simulink model "FullSystemNoFilters"  (R2023b)
settings: Solver=ode4  StartTime=0.0  StopTime=5  FixedStep=0.002  RelTol=1e-3  AbsTol=1e-6  EnableMultiTasking=on
undefined symbols (not defined in the file): den, kd, ki, kp, num, VMAX_DAC
settings Model: ExtModeTrigDuration=10000  Creator=MLevis  LastModifiedBy=JTayl
settings SolverCC: AutoScaleAbsTol=off  AlgebraicLoopSolver=TrustRegion  PositivePriorityOrder=on
settings DataIOCC: SaveFormat=Array  SignalLoggingSaveFormat=ModelDataLogs  ReturnWorkspaceOutputs=off
settings OptimizationCC: BlockReduction=off  BooleanDataType=off  OptimizeBlockIOStorage=off  BufferReuse=off  GlobalBufferReuse=off  ExpressionFolding=off  ExpressionDepthLimit=2147483647  LocalBlockOutputs=off  InitFltsAndDblsToZero=on  LifeSpan=inf  OptimizeDataStoreBuffers=off  BusAssignmentInplaceUpdate=off
settings DebuggingCC: SaveWithParameterizedLinksMsg=none  UnderspecifiedInitializationDetection=Classic  MergeDetectMultiDrivingBlocksExec=none  SignalResolutionControl=TryResolveAllWithWarning  MultiTaskDSMMsg=warning  MultiTaskCondExecSysMsg=none  FcnCallInpInsideContextMsg=warning  UnconnectedInputMsg=warning  UnconnectedOutputMsg=warning  UnconnectedLineMsg=warning  StateNameClashWarn=warning  SFUnexpectedBacktrackingDiag=warning  SFNoUnconditionalDefaultTransitionDiag=warning  SFExecutionAtInitializationDiag=none  ArithmeticOperatorsInVariantConditions=warning
settings HardwareCC: ProdBitPerPointer=32  ProdBitPerSizeT=32  ProdBitPerPtrDiffT=32  ProdLargestAtomicFloat=None  ProdIntDivRoundTo=Undefined  ProdEndianess=Unspecified  ProdWordSize=32  ProdHWDeviceType=32-bit Generic  TargetHWDeviceType=32-bit Generic
settings ModelReferenceCC: EnableRefExpFcnMdlSchedulingChecks=on  PropagateSignalLabelsOutOfModel=off
settings SFSimCC: CustomCodeUndefinedFunction=UseInterfaceOnly
settings RTWCC: Description=Quarc Win32 Target  SystemTargetFile=quarc_windows.tlc  TemplateMakefile=quarc_default_tmf
settings CodeAppCC: StateflowObjectComments=on
settings STFCustomTargetCC: TargetFcnLib=ansi_tfl_tmw.mat  TargetPreCompLibLocation=C:\PROGRA~3\QUARC\lib\2018b\windows\release  TargetLangStandard=C89/C90 (ANSI)  CPPClassGenCompliant=on  GRTInterface=on  SystemTargetFile=quarc_windows.tlc
settings GRTTargetCC: TargetFcnLib=ansi_tfl_tmw.mat  TargetPreCompLibLocation=C:\PROGRA~3\QUARC\lib\2018b\windows\release  TargetLangStandard=C89/C90 (ANSI)  ParMdlRefBuildCompliant=off  CompOptLevelCompliant=off  ConcurrentExecutionCompliant=off  CombineOutputUpdateFcns=off  MatFileLogging=off  GRTInterface=on  UseToolchainInfoCompliant=off  ExtMode=on  ExtModeMexFile=quarc_comm
settings ConfigComp: CovMetricSettings=dw  CovSaveCumulativeToWorkspaceVar=on  CovSaveSingleToWorkspaceVar=on

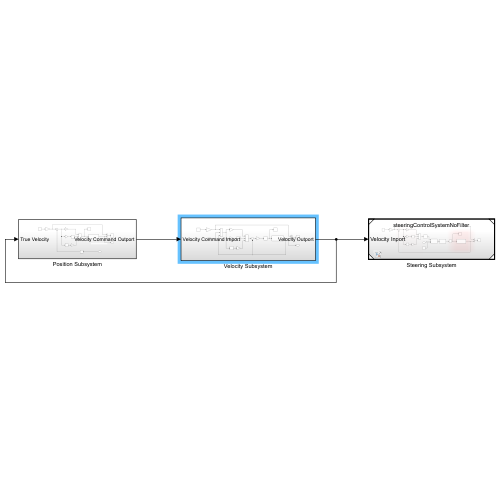
[thumbnail: Simulink's stored preview of the top-level diagram]
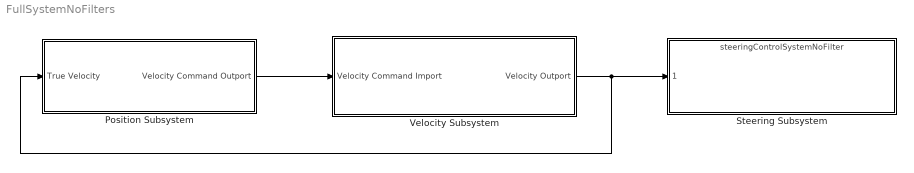
== system FullSystemNoFilters ==
  Position Subsystem : Subsystem
  Steering Subsystem : ModelReference  ModelNameDialog=steeringControlSystemNoFilter.slx  SimulationMode=Normal  ModelReferenceVersion=11.6
  Velocity Subsystem : Subsystem
  wires:
  Velocity Subsystem/1(Velocity Outport) -> Position Subsystem/1(True Velocity), Steering Subsystem/1
  Position Subsystem/1(Velocity Command Outport) -> Velocity Subsystem/1(Velocity Command Import)

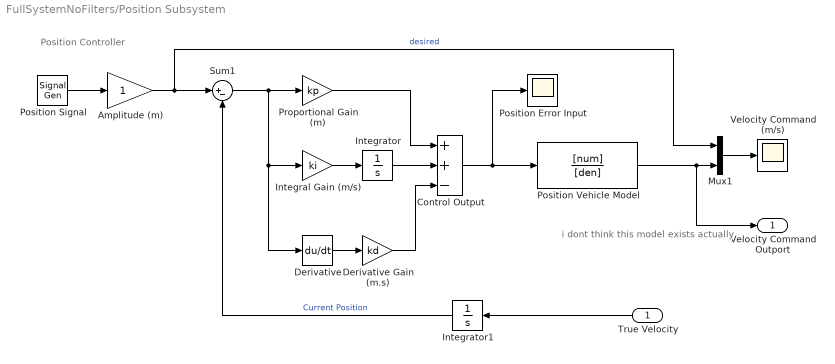
== system FullSystemNoFilters/Position Subsystem ==
  note: i dont think this model exists actually
  note: Position Controller
  True Velocity : Inport
  Amplitude (m) : Gain  SaturateOnIntegerOverflow=on  OutDataTypeStr=Inherit: Same as input  ParamDataTypeStr=Inherit: Same as input
  Control Output : Sum  Inputs=++-
  Derivative : Derivative
  Derivative Gain (m.s) : Gain  Gain=kd
  Integral Gain (m/s) : Gain  Gain=ki
  Integrator : Integrator  UpperSaturationLimit=VMAX_DAC  LowerSaturationLimit=-VMAX_DAC
  Integrator1 : Integrator
  Mux1 : Mux  Inputs=2
  Position Error Input : Scope
  Position Signal : SignalGenerator  Frequency=0.4  Units=rad/sec
  Position Vehicle Model : TransferFcn  Numerator=[num]  Denominator=[den]
  Proportional Gain (m) : Gain  Gain=kp
  Sum1 : Sum  Inputs=|+-
  Velocity Command (m/s) : Scope
  Velocity Command Outport : Outport
  wires:
  Sum1/1 -> Derivative/1, Integral Gain (m/s)/1, Proportional Gain (m)/1
  Position Vehicle Model/1 -> Velocity Command Outport/1, Mux1/2
  Control Output/1 -> Position Vehicle Model/1, Position Error Input/1
  Position Signal/1 -> Amplitude (m)/1
  Proportional Gain (m)/1 -> Control Output/1
  Amplitude (m)/1 -> Sum1/1, Mux1/1  "desired"
  Derivative Gain (m.s)/1 -> Control Output/3
  Integral Gain (m/s)/1 -> Integrator/1
  Derivative/1 -> Derivative Gain (m.s)/1
  Integrator/1 -> Control Output/2
  Mux1/1 -> Velocity Command (m/s)/1
  True Velocity/1 -> Integrator1/1
  Integrator1/1 -> Sum1/2  "Current Position"

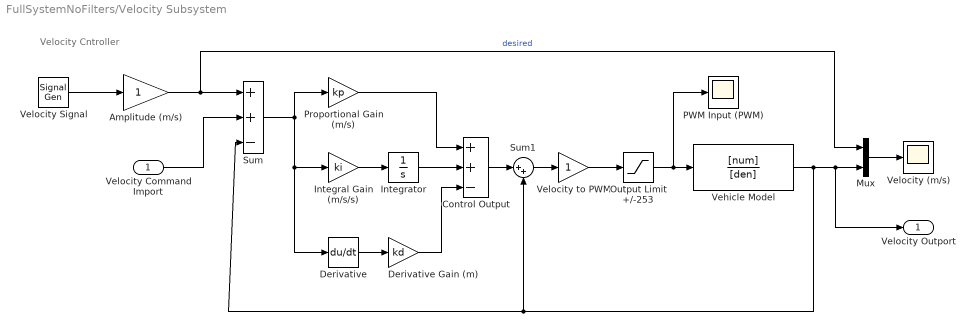
== system FullSystemNoFilters/Velocity Subsystem ==
  note: Velocity Cntroller
  Velocity Command Import : Inport
  Amplitude (m/s) : Gain  SaturateOnIntegerOverflow=on  OutDataTypeStr=Inherit: Same as input  ParamDataTypeStr=Inherit: Same as input
  Control Output : Sum  Inputs=++-
  Derivative : Derivative
  Derivative Gain (m) : Gain  Gain=kd
  Integral Gain (m/s/s) : Gain  Gain=ki
  Integrator : Integrator  UpperSaturationLimit=VMAX_DAC  LowerSaturationLimit=-VMAX_DAC
  Mux : Mux  Inputs=2
  "Output Limit +/-253 " : Saturate  UpperLimit=63  LowerLimit=-63
  PWM Input (PWM) : Scope
  Proportional Gain (m/s) : Gain  Gain=kp
  Sum : Sum  Inputs=++-
  Sum1 : Sum  Inputs=|++
  Vehicle Model : TransferFcn  Numerator=[num]  Denominator=[den]
  Velocity (m/s) : Scope
  Velocity Signal : SignalGenerator  Frequency=0.4  Units=rad/sec
  Velocity to PWM : Gain
  Velocity Outport : Outport
  wires:
  Velocity Signal/1 -> Amplitude (m/s)/1
  Amplitude (m/s)/1 -> Sum/1, Mux/1  "desired"
  Integrator/1 -> Control Output/2
  Vehicle Model/1 -> Sum/3, Sum1/2, Velocity Outport/1, Mux/2
  Mux/1 -> Velocity (m/s)/1
  Sum/1 -> Derivative/1, Integral Gain (m/s/s)/1, Proportional Gain (m/s)/1
  Integral Gain (m/s/s)/1 -> Integrator/1
  Derivative Gain (m)/1 -> Control Output/3
  "Output Limit +/-253 "/1 -> PWM Input (PWM)/1, Vehicle Model/1
  Velocity to PWM/1 -> "Output Limit +/-253 "/1
  Derivative/1 -> Derivative Gain (m)/1
  Proportional Gain (m/s)/1 -> Control Output/1
  Velocity Command Import/1 -> Sum/2
  Control Output/1 -> Sum1/1
  Sum1/1 -> Velocity to PWM/1
